simulink model "Messages4"  (R2020a)
settings: Solver=VariableStepAuto  StartTime=0.0  StopTime=0.3  RelTol=1e-3
settings Model: Creator=86188  LastModifiedBy=bzhan
settings DataIOCC: ReturnWorkspaceOutputs=off
settings DebuggingCC: ArithmeticOperatorsInVariantConditions=warning
settings SFSimCC: SimUseLocalCustomCode=off  CustomCodeUndefinedFunction=UseInterfaceOnly
settings RTWCC: RTWUseLocalCustomCode=off

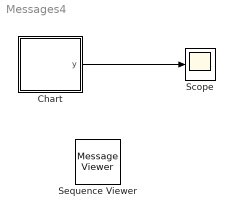
== system Messages4 ==
  Chart : Stateflow chart  TreatAsAtomicUnit=on
  Scope : Scope
  Sequence Viewer : MessageViewer
  wires:
  Chart/1(y) -> Scope/1

== stateflow chart Messages4/Chart ==
  settings: updateMethod=DISCRETE  sampleTime=0.1
  state A
    en:
    f("en_A");
    M.data=3;
    send(M);
  state B
    en:
    f("en_B");
    y=1;
  state C
    en:
    f("en_C");
    y=2;
  state D
    en:
    f("en_D");
    y=3;
  (default) -> A
  A -> B : M[M.data==3]
  B -> C : [M.data==3]
  C -> D : [M.data==4]
  data: s function_input; M local; y output
  function f(s):
    | function f(s)
    |   fprintf(s+"\n");
